simulink model "Modelo_Fuzzy_Manual"  (R2015b)
settings: Solver=ode1  StartTime=0.0  StopTime=tfin  FixedStep=0.05  RelTol=1e-5  AbsTol=1e-15
undefined symbols (not defined in the file): ACSP, ILSnoise, ParamFuzzy, wind
(part 2 of 2)

== system Modelo_Fuzzy_Manual/Main/A310 Model/Forces and Momments/Moments/Clmn/Cm/Fuzzy Cm1 (manual) ==
  q : Inport
  Va : Inport  Port=2
  Add : Sum
  Add1 : Sum
  CLa4 : Gain  Gain=ACSP.COEF.Cm.Cmq
  CLa5 : Gain  Gain=ACSP.MIG.Lref
  Constant : Constant  Value=ParamFuzzy.Cm1.min
  Constant1 : Constant  Value=ParamFuzzy.Cm1.max
  Membership function M : Subsystem
  Product : Product  Inputs=*/
  Product1 : Product  Inputs=**
  Product2 : Product  Inputs=**
  Product3 : Product  Inputs=*/
  Cm1 : Outport
  wires:
  q/1 -> Product/1
  Va/1 -> Product/2
  Product/1 -> Membership function M/1(q/Va)
  Membership function M/1(M1) -> Add1/1, Product1/2
  Membership function M/2(M2) -> Add1/2, Product2/1
  Constant/1 -> Product2/2
  Constant1/1 -> Product1/1
  Product2/1 -> Add/2
  Product1/1 -> Add/1
  Add/1 -> Product3/1
  Add1/1 -> Product3/2
  CLa5/1 -> CLa4/1
  Product3/1 -> CLa5/1
  CLa4/1 -> Cm1/1

== system Modelo_Fuzzy_Manual/Main/A310 Model/Forces and Momments/Moments/Clmn/Cm/Fuzzy Cm2 (manual) ==
  Hlg : Inport
  alpha : Inport  Port=2
  Constant1 : Constant  Value=0
  If Action Subsystem2 : Subsystem  TreatAsAtomicUnit=on
  If Action Subsystem3 : Subsystem  TreatAsAtomicUnit=on
  If1 : If  IfExpression=u1 > 40
  Sum2 : Sum  Inputs=|++
  Cm2 : Outport
  wires:
  If1/1 -> If Action Subsystem2/Action
  Constant1/1 -> If Action Subsystem2/1(In1)
  If Action Subsystem2/1(Out1) -> Sum2/1
  Sum2/1 -> Cm2/1
  If Action Subsystem3/1(CL2) -> Sum2/2
  Hlg/1 -> If Action Subsystem3/1(Hlg), If1/1
  alpha/1 -> If Action Subsystem3/2(alpha)
  If1/2 -> If Action Subsystem3/Action

== system Modelo_Fuzzy_Manual/Main/A310 Model/Forces and Momments/Moments/Clmn/Cn/Fuzzy Cn1 (manual) ==
  Va : Inport
  r : Inport  Port=2
  Add : Sum
  Add1 : Sum
  CLa4 : Gain  Gain=ACSP.COEF.Cn.Cnr
  CLa5 : Gain  Gain=ACSP.MIG.Lref
  Constant : Constant  Value=ParamFuzzy.Cn1.min
  Constant1 : Constant  Value=ParamFuzzy.Cn1.max
  Membership function M : Subsystem
  Product : Product  Inputs=*/
  Product1 : Product  Inputs=**
  Product2 : Product  Inputs=**
  Product3 : Product  Inputs=*/
  Cn1 : Outport
  wires:
  r/1 -> Product/1
  Va/1 -> Product/2
  Product/1 -> Membership function M/1(r/Va)
  Membership function M/1(M1) -> Add1/1, Product1/2
  Membership function M/2(M2) -> Add1/2, Product2/1
  Constant/1 -> Product2/2
  Constant1/1 -> Product1/1
  Product2/1 -> Add/2
  Product1/1 -> Add/1
  Add/1 -> Product3/1
  Add1/1 -> Product3/2
  CLa5/1 -> CLa4/1
  Product3/1 -> CLa5/1
  CLa4/1 -> Cn1/1

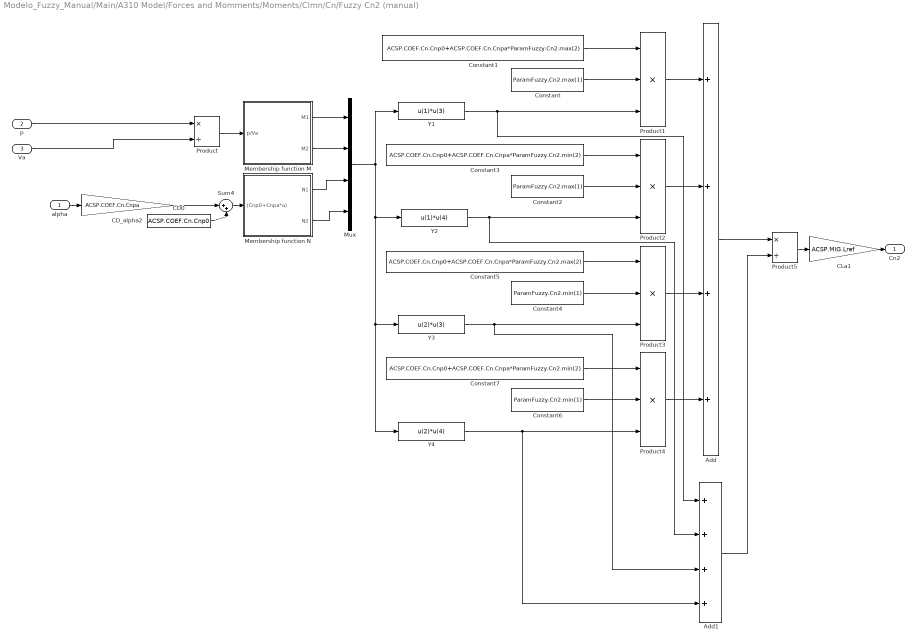
== system Modelo_Fuzzy_Manual/Main/A310 Model/Forces and Momments/Moments/Clmn/Cn/Fuzzy Cn2 (manual) ==
  alpha : Inport
  p : Inport  Port=2
  Va : Inport  Port=3
  Add : Sum  Inputs=++++
  Add1 : Sum  Inputs=++++
  CD0 : Constant  Value=ACSP.COEF.Cn.Cnp0
  CD_alpha2 : Gain  Gain=ACSP.COEF.Cn.Cnpa
  CLa1 : Gain  Gain=ACSP.MIG.Lref
  Constant : Constant  Value=ParamFuzzy.Cn2.max(1)
  Constant1 : Constant  Value=ACSP.COEF.Cn.Cnp0+ACSP.COEF.Cn.Cnpa*ParamFuzzy.Cn2.max(2)
  Constant2 : Constant  Value=ParamFuzzy.Cn2.max(1)
  Constant3 : Constant  Value=ACSP.COEF.Cn.Cnp0+ACSP.COEF.Cn.Cnpa*ParamFuzzy.Cn2.min(2)
  Constant4 : Constant  Value=ParamFuzzy.Cn2.min(1)
  Constant5 : Constant  Value=ACSP.COEF.Cn.Cnp0+ACSP.COEF.Cn.Cnpa*ParamFuzzy.Cn2.max(2)
  Constant6 : Constant  Value=ParamFuzzy.Cn2.min(1)
  Constant7 : Constant  Value=ACSP.COEF.Cn.Cnp0+ACSP.COEF.Cn.Cnpa*ParamFuzzy.Cn2.min(2)
  Membership function M : Subsystem
  Membership function N : Subsystem
  Mux : Mux
  Product : Product  Inputs=*/
  Product{1..4} (4 alike) : Product  Inputs=***
  Product5 : Product  Inputs=*/
  Sum4 : Sum  Inputs=|++
  Y1 : Fcn  Expr=u(1)*u(3)
  Y2 : Fcn  Expr=u(1)*u(4)
  Y3 : Fcn  Expr=u(2)*u(3)
  Y4 : Fcn  Expr=u(2)*u(4)
  Cn2 : Outport
  wires:
  ? -> ?
  p/1 -> Product/1
  Va/1 -> Product/2
  Product/1 -> Membership function M/1(p/Va)
  CD0/1 -> Sum4/2
  CD_alpha2/1 -> Sum4/1
  alpha/1 -> CD_alpha2/1
  Sum4/1 -> Membership function N/1((Cnp0+Cnpa*a))
  Membership function M/1(M1) -> Mux/1
  Membership function M/2(M2) -> Mux/2
  Membership function N/1(N1) -> Mux/3
  Membership function N/2(N2) -> Mux/4
  Mux/1 -> Y4/1, Y3/1, Y2/1, Y1/1
  Constant1/1 -> Product1/1
  Constant/1 -> Product1/2
  Y1/1 -> Add1/1, Product1/3
  Constant3/1 -> Product2/1
  Constant2/1 -> Product2/2
  Y2/1 -> Add1/2, Product2/3
  Constant5/1 -> Product3/1
  Constant4/1 -> Product3/2
  Y3/1 -> Add1/3, Product3/3
  Constant7/1 -> Product4/1
  Constant6/1 -> Product4/2
  Y4/1 -> Add1/4, Product4/3
  Product4/1 -> Add/4
  Product3/1 -> Add/3
  Product1/1 -> Add/1
  Product2/1 -> Add/2
  Add/1 -> Product5/1
  Add1/1 -> Product5/2
  Product5/1 -> CLa1/1
  CLa1/1 -> Cn2/1

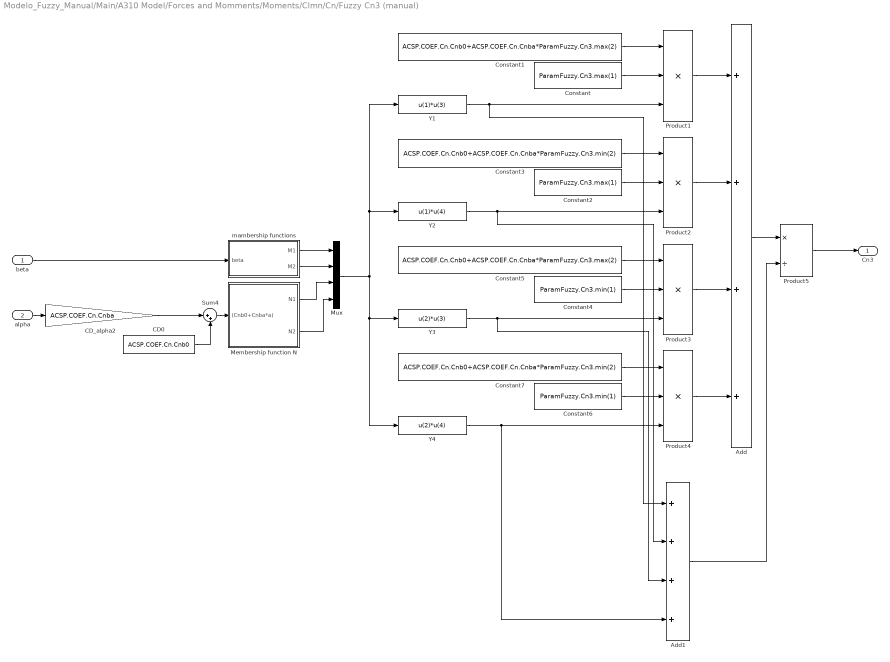
== system Modelo_Fuzzy_Manual/Main/A310 Model/Forces and Momments/Moments/Clmn/Cn/Fuzzy Cn3 (manual) ==
  beta : Inport
  alpha : Inport  Port=2
  Add : Sum  Inputs=++++
  Add1 : Sum  Inputs=++++
  CD0 : Constant  Value=ACSP.COEF.Cn.Cnb0
  CD_alpha2 : Gain  Gain=ACSP.COEF.Cn.Cnba
  Constant : Constant  Value=ParamFuzzy.Cn3.max(1)
  Constant1 : Constant  Value=ACSP.COEF.Cn.Cnb0+ACSP.COEF.Cn.Cnba*ParamFuzzy.Cn3.max(2)
  Constant2 : Constant  Value=ParamFuzzy.Cn3.max(1)
  Constant3 : Constant  Value=ACSP.COEF.Cn.Cnb0+ACSP.COEF.Cn.Cnba*ParamFuzzy.Cn3.min(2)
  Constant4 : Constant  Value=ParamFuzzy.Cn3.min(1)
  Constant5 : Constant  Value=ACSP.COEF.Cn.Cnb0+ACSP.COEF.Cn.Cnba*ParamFuzzy.Cn3.max(2)
  Constant6 : Constant  Value=ParamFuzzy.Cn3.min(1)
  Constant7 : Constant  Value=ACSP.COEF.Cn.Cnb0+ACSP.COEF.Cn.Cnba*ParamFuzzy.Cn3.min(2)
  Membership function N : Subsystem
  Mux : Mux
  Product{1..4} (4 alike) : Product  Inputs=***
  Product5 : Product  Inputs=*/
  Sum4 : Sum  Inputs=|++
  Y1 : Fcn  Expr=u(1)*u(3)
  Y2 : Fcn  Expr=u(1)*u(4)
  Y3 : Fcn  Expr=u(2)*u(3)
  Y4 : Fcn  Expr=u(2)*u(4)
  mambership functions : Subsystem
  Cn3 : Outport
  wires:
  beta/1 -> mambership functions/1(beta)
  CD0/1 -> Sum4/2
  CD_alpha2/1 -> Sum4/1
  Sum4/1 -> Membership function N/1((Cnb0+Cnba*a))
  alpha/1 -> CD_alpha2/1
  mambership functions/1(M1) -> Mux/1
  mambership functions/2(M2) -> Mux/2
  Membership function N/1(N1) -> Mux/3
  Membership function N/2(N2) -> Mux/4
  Mux/1 -> Y4/1, Y3/1, Y1/1, Y2/1
  Constant/1 -> Product1/2
  Y1/1 -> Add1/1, Product1/3
  Constant1/1 -> Product1/1
  Constant2/1 -> Product2/2
  Constant3/1 -> Product2/1
  Y2/1 -> Add1/2, Product2/3
  Constant4/1 -> Product3/2
  Constant5/1 -> Product3/1
  Y3/1 -> Add1/3, Product3/3
  Constant6/1 -> Product4/2
  Constant7/1 -> Product4/1
  Y4/1 -> Add1/4, Product4/3
  Product1/1 -> Add/1
  Product2/1 -> Add/2
  Product3/1 -> Add/3
  Product4/1 -> Add/4
  Add/1 -> Product5/1
  Product5/1 -> Cn3/1
  Add1/1 -> Product5/2

== system Modelo_Fuzzy_Manual/Main/A310 Model/Forces and Momments/Forces/CXYZ/Fuzzy CL2 (manual)/If Action Subsystem1/membership function M ==
  Hlg : Inport
  Abs : Abs
  CLa1 : Gain  Gain=ACSP.COEF.CL.lambdah
  Constant : Constant
  Constant1 : Constant
  Constant2 : Constant  Value=1/(2*ParamFuzzy.CL2.max)
  Constant3 : Constant
  Gain2 : Gain  Gain=-1
  Math Function : Math  SaturateOnIntegerOverflow=on
  Product : Product  Inputs=*/
  Product1 : Product  Inputs=**
  Product2 : Product  Inputs=**
  Sum : Sum  Inputs=|+-
  Sum1 : Sum  Inputs=|++
  Sum2 : Sum  Inputs=|+-
  Sum3 : Sum  Inputs=-+|
  M1 : Outport
  M2 : Outport  Port=2
  wires:
  Abs/1 -> Product1/1, Sum1/2, Gain2/1
  Gain2/1 -> Math Function/1
  CLa1/1 -> Abs/1
  Hlg/1 -> Product2/2, CLa1/1
  Math Function/1 -> Sum/1
  Constant/1 -> Sum/2
  Sum/1 -> Sum1/1
  Sum1/1 -> Product/1
  Product/1 -> Sum3/1, M1/1
  Product1/1 -> Product/2
  Constant1/1 -> Sum2/1
  Sum2/1 -> Product1/2
  Product2/1 -> Sum2/2
  Constant2/1 -> Product2/1
  Sum3/1 -> M2/1
  Constant3/1 -> Sum3/2

== system Modelo_Fuzzy_Manual/Main/A310 Model/Forces and Momments/Moments/Clmn/Cl/Fuzzy Cl1 (manual)/Membership function M ==
  p/Va : Inport
  Constant : Constant  Value=ParamFuzzy.Cl1.min
  Constant1 : Constant  Value=ParamFuzzy.Cl1.max
  Constant2 : Constant
  Product : Product  Inputs=*/
  Sum : Sum  Inputs=|+-
  Sum1 : Sum  Inputs=|-+
  Sum2 : Sum  Inputs=-+
  M1 : Outport
  M2 : Outport  Port=2
  wires:
  p/Va/1 -> Sum/1
  Constant/1 -> Sum1/1, Sum/2
  Sum/1 -> Product/1
  Sum1/1 -> Product/2
  Constant1/1 -> Sum1/2
  Product/1 -> Sum2/1, M1/1
  Constant2/1 -> Sum2/2
  Sum2/1 -> M2/1

== system Modelo_Fuzzy_Manual/Main/A310 Model/Forces and Momments/Moments/Clmn/Cl/Fuzzy Cl2 (manual)/Membership function M ==
  p/Va : Inport
  Constant : Constant  Value=ParamFuzzy.Cl2.min(1)
  Constant1 : Constant  Value=ParamFuzzy.Cl2.max(1)
  Constant2 : Constant
  Product : Product  Inputs=*/
  Sum : Sum  Inputs=|+-
  Sum1 : Sum  Inputs=|-+
  Sum2 : Sum  Inputs=-+
  M1 : Outport
  M2 : Outport  Port=2
  wires:
  p/Va/1 -> Sum/1
  Constant/1 -> Sum1/1, Sum/2
  Sum/1 -> Product/1
  Sum1/1 -> Product/2
  Constant1/1 -> Sum1/2
  Product/1 -> Sum2/1, M1/1
  Constant2/1 -> Sum2/2
  Sum2/1 -> M2/1

== system Modelo_Fuzzy_Manual/Main/A310 Model/Forces and Momments/Moments/Clmn/Cl/Fuzzy Cl2 (manual)/Membership function N ==
  (Clr0+Clra*a) : Inport
  Constant : Constant  Value=ACSP.COEF.Cl.Clr0+ACSP.COEF.Cl.Clra*ParamFuzzy.Cl2.min(2)
  Constant1 : Constant  Value=ACSP.COEF.Cl.Clr0+ACSP.COEF.Cl.Clra*ParamFuzzy.Cl2.max(2)
  Constant2 : Constant
  Product : Product  Inputs=*/
  Sum : Sum  Inputs=|+-
  Sum1 : Sum  Inputs=|-+
  Sum2 : Sum  Inputs=-+
  N1 : Outport
  N2 : Outport  Port=2
  wires:
  (Clr0+Clra*a)/1 -> Sum/1
  Constant/1 -> Sum1/1, Sum/2
  Sum1/1 -> Product/2
  Sum/1 -> Product/1
  Constant1/1 -> Sum1/2
  Product/1 -> Sum2/1, N1/1
  Constant2/1 -> Sum2/2
  Sum2/1 -> N2/1

== system Modelo_Fuzzy_Manual/Main/A310 Model/Forces and Momments/Moments/Clmn/Cm/Fuzzy Cm1 (manual)/Membership function M ==
  q/Va : Inport
  Constant : Constant  Value=ParamFuzzy.Cm1.min
  Constant1 : Constant  Value=ParamFuzzy.Cm1.max
  Constant2 : Constant
  Product : Product  Inputs=*/
  Sum : Sum  Inputs=|+-
  Sum1 : Sum  Inputs=|-+
  Sum2 : Sum  Inputs=-+
  M1 : Outport
  M2 : Outport  Port=2
  wires:
  q/Va/1 -> Sum/1
  Constant/1 -> Sum1/1, Sum/2
  Sum/1 -> Product/1
  Sum1/1 -> Product/2
  Constant1/1 -> Sum1/2
  Product/1 -> Sum2/1, M1/1
  Constant2/1 -> Sum2/2
  Sum2/1 -> M2/1

== system Modelo_Fuzzy_Manual/Main/A310 Model/Forces and Momments/Moments/Clmn/Cm/Fuzzy Cm2 (manual)/If Action Subsystem2 ==
  In1 : Inport
  Action Port : ActionPort  InitializeStates=reset  ActionType=then
  Out1 : Outport
  wires:
  In1/1 -> Out1/1

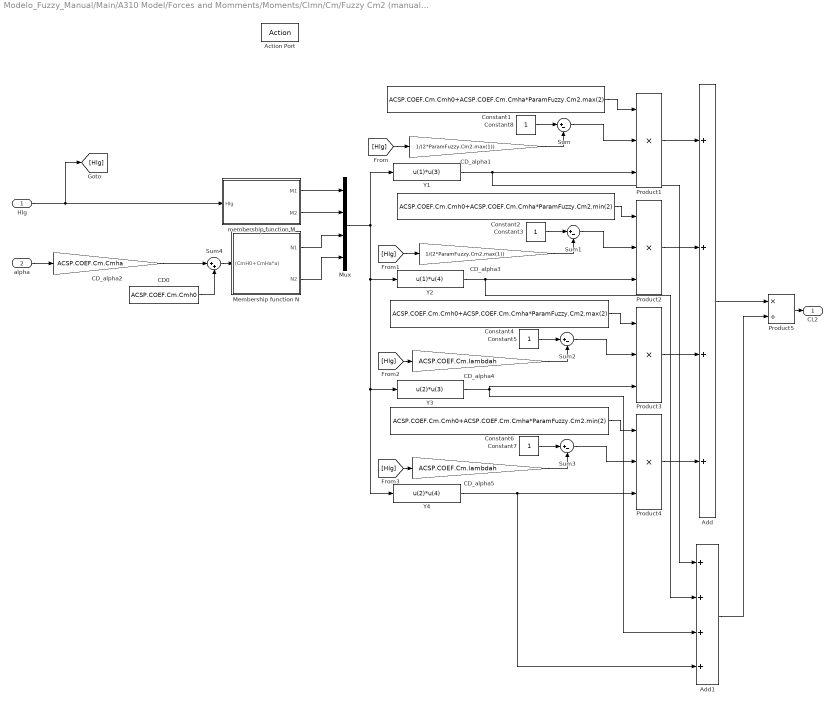
== system Modelo_Fuzzy_Manual/Main/A310 Model/Forces and Momments/Moments/Clmn/Cm/Fuzzy Cm2 (manual)/If Action Subsystem3 ==
  Hlg : Inport
  alpha : Inport  Port=2
  Action Port : ActionPort  ActionType=else
  Add : Sum  Inputs=++++
  Add1 : Sum  Inputs=++++
  CD0 : Constant  Value=ACSP.COEF.Cm.Cmh0
  CD_alpha1 : Gain  Gain=1/(2*ParamFuzzy.Cm2.max(1))
  CD_alpha2 : Gain  Gain=ACSP.COEF.Cm.Cmha
  CD_alpha3 : Gain  Gain=1/(2*ParamFuzzy.Cm2.max(1))
  CD_alpha4 : Gain  Gain=ACSP.COEF.Cm.lambdah
  CD_alpha5 : Gain  Gain=ACSP.COEF.Cm.lambdah
  Constant1 : Constant  Value=ACSP.COEF.Cm.Cmh0+ACSP.COEF.Cm.Cmha*ParamFuzzy.Cm2.max(2)
  Constant2 : Constant  Value=ACSP.COEF.Cm.Cmh0+ACSP.COEF.Cm.Cmha*ParamFuzzy.Cm2.min(2)
  Constant{3,5,7..8} (4 alike) : Constant
  Constant4 : Constant  Value=ACSP.COEF.Cm.Cmh0+ACSP.COEF.Cm.Cmha*ParamFuzzy.Cm2.max(2)
  Constant6 : Constant  Value=ACSP.COEF.Cm.Cmh0+ACSP.COEF.Cm.Cmha*ParamFuzzy.Cm2.min(2)
  Membership function N : Subsystem
  Mux : Mux
  Product{1..4} (4 alike) : Product  Inputs=***
  Product5 : Product  Inputs=*/
  Sum{,1..3} (4 alike) : Sum  Inputs=|+-
  Sum4 : Sum  Inputs=|++
  Y1 : Fcn  Expr=u(1)*u(3)
  Y2 : Fcn  Expr=u(1)*u(4)
  Y3 : Fcn  Expr=u(2)*u(3)
  Y4 : Fcn  Expr=u(2)*u(4)
  membership function M : Subsystem
  CL2 : Outport
  wires:
  Hlg/1 -> [Hlg], membership function M/1(Hlg)
  CD0/1 -> Sum4/2
  CD_alpha2/1 -> Sum4/1
  Sum4/1 -> Membership function N/1((CmH0+CmHa*a))
  alpha/1 -> CD_alpha2/1
  membership function M/1(M1) -> Mux/1
  membership function M/2(M2) -> Mux/2
  Membership function N/1(N1) -> Mux/3
  Membership function N/2(N2) -> Mux/4
  Mux/1 -> Y4/1, Y3/1, Y2/1, Y1/1
  Y1/1 -> Add1/1, Product1/3
  Y2/1 -> Add1/2, Product2/3
  Y3/1 -> Product3/3, Add1/3
  Y4/1 -> Add1/4, Product4/3
  Product4/1 -> Add/4
  Product3/1 -> Add/3
  Product1/1 -> Add/1
  Product2/1 -> Add/2
  Add/1 -> Product5/1
  Add1/1 -> Product5/2
  Product5/1 -> CL2/1
  Constant8/1 -> Sum/1
  [Hlg] -> CD_alpha1/1
  CD_alpha1/1 -> Sum/2
  Sum/1 -> Product1/2
  Constant1/1 -> Product1/1
  Constant3/1 -> Sum1/1
  [Hlg] -> CD_alpha3/1
  CD_alpha3/1 -> Sum1/2
  Sum1/1 -> Product2/2
  Constant2/1 -> Product2/1
  Constant5/1 -> Sum2/1
  [Hlg] -> CD_alpha4/1
  CD_alpha4/1 -> Sum2/2
  Sum2/1 -> Product3/2
  Constant4/1 -> Product3/1
  Constant7/1 -> Sum3/1
  [Hlg] -> CD_alpha5/1
  CD_alpha5/1 -> Sum3/2
  Sum3/1 -> Product4/2
  Constant6/1 -> Product4/1

== system Modelo_Fuzzy_Manual/Main/A310 Model/Forces and Momments/Moments/Clmn/Cn/Fuzzy Cn1 (manual)/Membership function M ==
  r/Va : Inport
  Constant : Constant  Value=ParamFuzzy.Cn1.min
  Constant1 : Constant  Value=ParamFuzzy.Cn1.max
  Constant2 : Constant
  Product : Product  Inputs=*/
  Sum : Sum  Inputs=|+-
  Sum1 : Sum  Inputs=|-+
  Sum2 : Sum  Inputs=-+
  M1 : Outport
  M2 : Outport  Port=2
  wires:
  r/Va/1 -> Sum/1
  Constant/1 -> Sum1/1, Sum/2
  Sum/1 -> Product/1
  Sum1/1 -> Product/2
  Constant1/1 -> Sum1/2
  Product/1 -> Sum2/1, M1/1
  Constant2/1 -> Sum2/2
  Sum2/1 -> M2/1

== system Modelo_Fuzzy_Manual/Main/A310 Model/Forces and Momments/Moments/Clmn/Cn/Fuzzy Cn2 (manual)/Membership function M ==
  p/Va : Inport
  Constant : Constant  Value=ParamFuzzy.Cn2.min(1)
  Constant1 : Constant  Value=ParamFuzzy.Cn2.max(1)
  Constant2 : Constant
  Product : Product  Inputs=*/
  Sum : Sum  Inputs=|+-
  Sum1 : Sum  Inputs=|-+
  Sum2 : Sum  Inputs=-+
  M1 : Outport
  M2 : Outport  Port=2
  wires:
  p/Va/1 -> Sum/1
  Constant/1 -> Sum1/1, Sum/2
  Sum/1 -> Product/1
  Sum1/1 -> Product/2
  Constant1/1 -> Sum1/2
  Product/1 -> Sum2/1, M1/1
  Constant2/1 -> Sum2/2
  Sum2/1 -> M2/1

== system Modelo_Fuzzy_Manual/Main/A310 Model/Forces and Momments/Moments/Clmn/Cn/Fuzzy Cn2 (manual)/Membership function N ==
  (Cnp0+Cnpa*a) : Inport
  Constant : Constant  Value=ACSP.COEF.Cn.Cnp0+ACSP.COEF.Cn.Cnpa*ParamFuzzy.Cn2.min(2)
  Constant1 : Constant  Value=ACSP.COEF.Cn.Cnp0+ACSP.COEF.Cn.Cnpa*ParamFuzzy.Cn2.max(2)
  Constant2 : Constant
  Product : Product  Inputs=*/
  Sum : Sum  Inputs=|+-
  Sum1 : Sum  Inputs=|-+
  Sum2 : Sum  Inputs=-+
  N1 : Outport
  N2 : Outport  Port=2
  wires:
  (Cnp0+Cnpa*a)/1 -> Sum/1
  Constant/1 -> Sum1/1, Sum/2
  Sum1/1 -> Product/2
  Sum/1 -> Product/1
  Constant1/1 -> Sum1/2
  Product/1 -> Sum2/1, N1/1
  Constant2/1 -> Sum2/2
  Sum2/1 -> N2/1

== system Modelo_Fuzzy_Manual/Main/A310 Model/Forces and Momments/Moments/Clmn/Cn/Fuzzy Cn3 (manual)/Membership function N ==
  (Cnb0+Cnba*a) : Inport
  Constant : Constant  Value=ACSP.COEF.Cn.Cnb0+ACSP.COEF.Cn.Cnba*ParamFuzzy.Cn3.min(2)
  Constant1 : Constant  Value=ACSP.COEF.Cn.Cnb0+ACSP.COEF.Cn.Cnba*ParamFuzzy.Cn3.max(2)
  Constant2 : Constant
  Product : Product  Inputs=*/
  Sum : Sum  Inputs=|+-
  Sum1 : Sum  Inputs=|-+
  Sum2 : Sum  Inputs=-+
  N1 : Outport
  N2 : Outport  Port=2
  wires:
  (Cnb0+Cnba*a)/1 -> Sum/1
  Constant/1 -> Sum1/1, Sum/2
  Sum1/1 -> Product/2
  Sum/1 -> Product/1
  Constant1/1 -> Sum1/2
  Product/1 -> Sum2/1, N1/1
  Constant2/1 -> Sum2/2
  Sum2/1 -> N2/1

== system Modelo_Fuzzy_Manual/Main/A310 Model/Forces and Momments/Moments/Clmn/Cn/Fuzzy Cn3 (manual)/mambership functions ==
  beta : Inport
  Constant : Constant  Value=ParamFuzzy.Cn3.max(1)
  Constant1 : Constant
  Gain : Gain  Gain=1/(2*ParamFuzzy.Cn3.max(1))
  Sum : Sum  Inputs=|++
  Sum1 : Sum  Inputs=|-+
  M1 : Outport
  M2 : Outport  Port=2
  wires:
  beta/1 -> Sum/1
  Constant/1 -> Sum/2
  Sum/1 -> Gain/1
  Gain/1 -> Sum1/1, M1/1
  Constant1/1 -> Sum1/2
  Sum1/1 -> M2/1

== system Modelo_Fuzzy_Manual/Main/A310 Model/Forces and Momments/Moments/Clmn/Cm/Fuzzy Cm2 (manual)/If Action Subsystem3/Membership function N ==
  (CmH0+CmHa*a) : Inport
  Constant : Constant  Value=ACSP.COEF.Cm.Cmh0+ACSP.COEF.Cm.Cmha*ParamFuzzy.Cm2.min(2)
  Constant1 : Constant  Value=ACSP.COEF.Cm.Cmh0+ACSP.COEF.Cm.Cmha*ParamFuzzy.Cm2.max(2)
  Constant2 : Constant
  Product : Product  Inputs=*/
  Sum : Sum  Inputs=|+-
  Sum1 : Sum  Inputs=|-+
  Sum2 : Sum  Inputs=-+
  N1 : Outport
  N2 : Outport  Port=2
  wires:
  (CmH0+CmHa*a)/1 -> Sum/1
  Constant/1 -> Sum1/1, Sum/2
  Sum1/1 -> Product/2
  Sum/1 -> Product/1
  Constant1/1 -> Sum1/2
  Product/1 -> Sum2/1, N1/1
  Constant2/1 -> Sum2/2
  Sum2/1 -> N2/1

== system Modelo_Fuzzy_Manual/Main/A310 Model/Forces and Momments/Moments/Clmn/Cm/Fuzzy Cm2 (manual)/If Action Subsystem3/membership function M ==
  Hlg : Inport
  Abs : Abs
  CLa1 : Gain  Gain=ACSP.COEF.Cm.lambdah
  Constant : Constant
  Constant1 : Constant
  Constant2 : Constant  Value=1/(2*ParamFuzzy.Cm2.max(1))
  Constant3 : Constant
  Gain2 : Gain  Gain=-1
  Math Function : Math  SaturateOnIntegerOverflow=on
  Product : Product  Inputs=*/
  Product1 : Product  Inputs=**
  Product2 : Product  Inputs=**
  Sum : Sum  Inputs=|+-
  Sum1 : Sum  Inputs=|++
  Sum2 : Sum  Inputs=|+-
  Sum3 : Sum  Inputs=-+|
  M1 : Outport
  M2 : Outport  Port=2
  wires:
  Abs/1 -> Product1/1, Sum1/2, Gain2/1
  Gain2/1 -> Math Function/1
  CLa1/1 -> Abs/1
  Hlg/1 -> Product2/2, CLa1/1
  Math Function/1 -> Sum/1
  Constant/1 -> Sum/2
  Sum/1 -> Sum1/1
  Sum1/1 -> Product/1
  Product/1 -> Sum3/1, M1/1
  Product1/1 -> Product/2
  Constant1/1 -> Sum2/1
  Sum2/1 -> Product1/2
  Product2/1 -> Sum2/2
  Constant2/1 -> Product2/1
  Sum3/1 -> M2/1
  Constant3/1 -> Sum3/2
